simulink model "task_2_alpha05_mu_u"  (R2021b)
settings: Solver=FixedStepAuto  StartTime=0.0  StopTime=12  FixedStep=0.00005  RelTol=1e-3
settings Model: Creator=den  LastModifiedBy=den

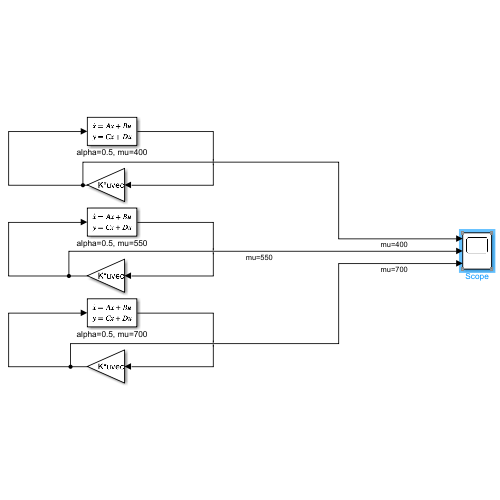
[thumbnail: Simulink's stored preview of the top-level diagram]
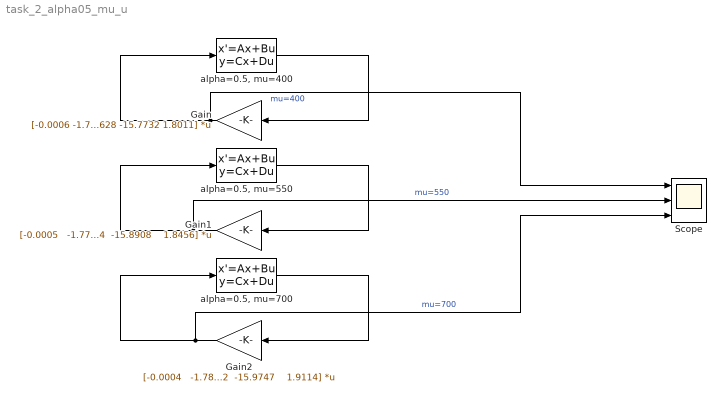
== system task_2_alpha05_mu_u ==
  Gain : Gain  Gain=[-0.0006 -1.7628 -15.7732 1.8011]  Multiplication=Matrix(K*u) (u vector)
  Gain1 : Gain  Gain="[-0.0005   -1.7764  -15.8908    1.8456]"  Multiplication=Matrix(K*u) (u vector)
  Gain2 : Gain  Gain="[-0.0004   -1.7882  -15.9747    1.9114]"  Multiplication=Matrix(K*u) (u vector)
  Scope : Scope  NumInputPorts=3
  "alpha=0.5, mu=400" : StateSpace  A=[-3 0 0 0; 0 3 0 0; 0 0 3 3; 0 0 -3 3]  B=[0; 7; 0; 1]  C=[1 0 0 0; 0 1 0 0; 0 0 1 0; 0 0 0 1]  D=[0; 0; 0; 0]  InitialCondition=[-3; 17; 2; -8]
  "alpha=0.5, mu=550" : StateSpace  A=[-3 0 0 0; 0 3 0 0; 0 0 3 3; 0 0 -3 3]  B=[0; 7; 0; 1]  C=[1 0 0 0; 0 1 0 0; 0 0 1 0; 0 0 0 1]  D=[0; 0; 0; 0]  InitialCondition=[-3; 17; 2; -8]
  "alpha=0.5, mu=700" : StateSpace  A=[-3 0 0 0; 0 3 0 0; 0 0 3 3; 0 0 -3 3]  B=[0; 7; 0; 1]  C=[1 0 0 0; 0 1 0 0; 0 0 1 0; 0 0 0 1]  D=[0; 0; 0; 0]  InitialCondition=[-3; 17; 2; -8]
  wires:
  "alpha=0.5, mu=400"/1 -> Gain/1
  Gain/1 -> Scope/1, "alpha=0.5, mu=400"/1  "mu=400"
  Gain1/1 -> Scope/2, "alpha=0.5, mu=550"/1  "mu=550"
  "alpha=0.5, mu=550"/1 -> Gain1/1
  Gain2/1 -> Scope/3, "alpha=0.5, mu=700"/1  "mu=700"
  "alpha=0.5, mu=700"/1 -> Gain2/1
